simulink model "DCmotor"  (R2024a)
settings: Solver=VariableStepAuto  StartTime=0.0  StopTime=10.0  RelTol=1e-3
libraries: dspfdesign x1
settings Model: Creator=dcrea  LastModifiedBy=dcrea

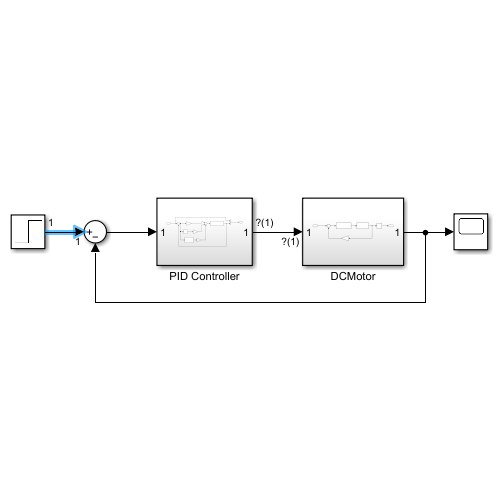
[thumbnail: Simulink's stored preview of the top-level diagram]
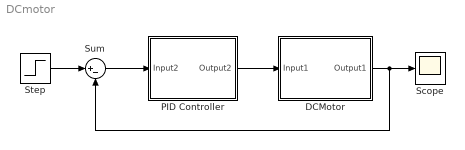
== system DCmotor ==
  DCMotor : Subsystem
  PID Controller : Subsystem
  Scope : Scope
  Step : Step  SampleTime=0
  Sum : Sum  Inputs=|+-
  wires:
  Sum/1 -> PID Controller/1(Input2)
  Step/1 -> Sum/1
  DCMotor/1(Output1) -> Scope/1, Sum/2
  PID Controller/1(Output2) -> DCMotor/1(Input1)

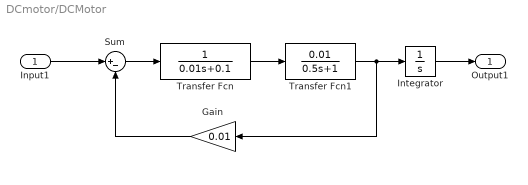
== system DCmotor/DCMotor ==
  Input1 : Inport
  Gain : Gain  Gain=0.01
  Integrator : Integrator
  Sum : Sum  Inputs=|+-
  Transfer Fcn : TransferFcn  Denominator=[0.01 0.1]
  Transfer Fcn1 : TransferFcn  Numerator=[0.01]  Denominator=[0.5 1]
  Output1 : Outport
  wires:
  Input1/1 -> Sum/1
  Transfer Fcn/1 -> Transfer Fcn1/1
  Gain/1 -> Sum/2
  Sum/1 -> Transfer Fcn/1
  Integrator/1 -> Output1/1
  Transfer Fcn1/1 -> Gain/1, Integrator/1

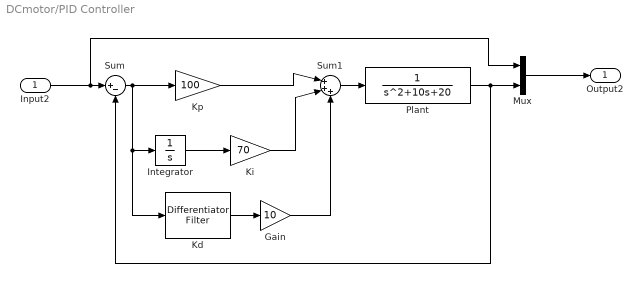
== system DCmotor/PID Controller ==
  Input2 : Inport
  Gain : Gain  Gain=10
  Integrator : Integrator
  Kd : dspfdesign/Differentiator Filter  DesignForMinimumOrder=on  FilterOrder=31  PassbandRipple=0.1  ScaleCoefficients=off  SimulateUsing=Interpreted execution  roundingMode=Floor  coeffsDataTypeStr=fixdt(1,16)
  Ki : Gain  Gain=70
  Kp : Gain  Gain=100
  Mux : Mux  Inputs=2
  Plant : TransferFcn  Denominator=[1 10 20]
  Sum : Sum  Inputs=|+-
  Sum1 : Sum  Inputs=|+++
  Output2 : Outport
  wires:
  Plant/1 -> Mux/2, Sum/2
  Kp/1 -> Sum1/1
  Ki/1 -> Sum1/2
  Input2/1 -> Mux/1, Sum/1
  Sum/1 -> Kd/1, Integrator/1, Kp/1
  Kd/1 -> Gain/1
  Mux/1 -> Output2/1
  Sum1/1 -> Plant/1
  Gain/1 -> Sum1/3
  Integrator/1 -> Ki/1
